simulink model "hand_assembly_3test"  (R2024b)
settings: Solver=daessc  StartTime=0.0  StopTime=10.0  RelTol=1e-3
values from neighbouring files (symbols this model uses):
  Ix1 = 0.000555447536833    [C6_workspace.mat]
  Ix2 = 0.000647276077146    [C6_workspace.mat]
  Ix3 = 0.000647276077146    [C6_workspace.mat]
  Ix4 = 0.00061268668168    [C6_workspace.mat]
  Iy1 = 0.000281297083333    [C6_workspace.mat]
  Iy2 = 0.000285516539583    [C6_workspace.mat]
  Iy3 = 0.000285516539583    [C6_workspace.mat]
  Iy4 = 0.000286923025    [C6_workspace.mat]
  Iz1 = 0.000673203786833    [C6_workspace.mat]
  Iz2 = 0.000766798670896    [C6_workspace.mat]
  Iz3 = 0.000766798670896    [C6_workspace.mat]
  Iz4 = 0.00073279805668    [C6_workspace.mat]
  m_1 = 0.245    [C6_workspace.mat]
  m_2 = 0.275    [C6_workspace.mat]
  m_3 = 0.275    [C6_workspace.mat]
  m_4 = 0.285    [C6_workspace.mat]
undefined symbols (not defined in the file or in its folder): X, Y, Z
libraries: sm_lib x115, nesl_utility x25, robotcorelib x3
(part 7 of 8)

== matlab function hand_assembly_3test/Dynamics finger 3 ==
  data: theta input size=[4,1]; tau output size=[4,1]; thetad input size=[4,1]; thetadd input size=[4,1]; thetaref input size=[4,1]; thetarefd input size=[4,1]; thetarefdd input size=[4,1]; Kp input; Kd input
function tau  = dynamics(theta, thetad, thetadd, thetaref, thetarefd, thetarefdd, Kp, Kd)
%defining parameters
m_1 = 2; 
m_2 = 2.03;
m_3 = 2.03;
m_4 = 2.04;
a_1 = 0.053311;
L_2 = 0.057755;
L_3 = 0.057755;
L_4 = 0.055798;
%d_1 = 0.04288;
w_1 = 0.03460;
w_2 = 0.03460;
w_3 = 0.03460;
w_4 = 0.03460;
h_1 = 0.02215;
h_2 = 0.02215;
h_3 = 0.02215;
h_4 = 0.02215;

%defining inputs

theta_1 = theta(1);
theta_2 = theta(2);
theta_3 = theta(3);
theta_4 = theta(4);
thetad_1 = thetad(1);
thetad_2 = thetad(2);
thetad_3 = thetad(3);
thetad_4 = thetad(4);
thetad = [thetad_1; thetad_2; thetad_3; thetad_4];

thetadd_1 = thetadd(1);
thetadd_2 = thetadd(2);
thetadd_3 = thetadd(3);
thetadd_4 = thetadd(4);
thetadd = [thetadd_1; thetadd_2; thetadd_3; thetadd_4];

thetaref_1 = thetaref(1);
thetaref_2 = thetaref(2);
thetaref_3 = thetaref(3);
thetaref_4 = thetaref(4);
thetaref = [thetaref_1; thetaref_2; thetaref_3; thetaref_4];

thetarefd_1 = thetarefd(1);
thetarefd_2 = thetarefd(2);
thetarefd_3 = thetarefd(3);
thetarefd_4 = thetarefd(4);
thetarefd = [thetarefd_1; thetarefd_2; thetarefd_3; thetarefd_4];

thetarefdd_1 = thetarefdd(1);
thetarefdd_2 = thetarefdd(2);
thetarefdd_3 = thetarefdd(3);
thetarefdd_4 = thetarefdd(4);
thetarefdd = [thetarefdd_1; thetarefdd_2; thetarefdd_3; thetarefdd_4];

thetaE = thetaref - theta;
thetaEd = thetarefd - thetad;



%%%%%%%%%%%%%%%%%%%%%%%%%%%%%%%%%%%%%%%%%%%%%%%%%%%%%%%%%%%%%%%%%%%%%%%%%%%%%%%defining inertia matrix M

M11= (1/12)*m_1*(a_1^2 + h_1^2) + (1/12)*m_2*(L_2^2 + h_2^2) + m_2*(L_2*cos(theta_2) + L_3*cos(theta_2 + theta_3) + L_4*cos(theta_2 + theta_3 + theta_4) + a_1)^2*sin(theta_1)^2 + (1/12)*m_3*(L_3^2 + h_3^2) + m_3*(L_2*cos(theta_2) + L_3*cos(theta_2 + theta_3) + L_4*cos(theta_2 + theta_3 + theta_4) + a_1)^2*cos(theta_1)^2 + (1/12)*m_4*(L_4^2 + h_4^2);
M12 = -m_2*(-L_2*sin(theta_2) - L_3*sin(theta_2 + theta_3) - L_4*sin(theta_2 + theta_3 + theta_4))*(L_2*cos(theta_2) + L_3*cos(theta_2 + theta_3) + L_4*cos(theta_2 + theta_3 + theta_4) + a_1)*sin(theta_1)*cos(theta_1) + m_3*(-L_2*sin(theta_2) - L_3*sin(theta_2 + theta_3) - L_4*sin(theta_2 + theta_3 + theta_4))*(L_2*cos(theta_2) + L_3*cos(theta_2 + theta_3) + L_4*cos(theta_2 + theta_3 + theta_4) + a_1)*sin(theta_1)*cos(theta_1);

M13 = -m_2*(-L_3*sin(theta_2 + theta_3) - L_4*sin(theta_2 + theta_3 + theta_4))*(L_2*cos(theta_2) + L_3*cos(theta_2 + theta_3) + L_4*cos(theta_2 + theta_3 + theta_4) + a_1)*sin(theta_1)*cos(theta_1) + m_3*(-L_3*sin(theta_2 + theta_3) - L_4*sin(theta_2 + theta_3 + theta_4))*(L_2*cos(theta_2) + L_3*cos(theta_2 + theta_3) + L_4*cos(theta_2 + theta_3 + theta_4) + a_1)*sin(theta_1)*cos(theta_1);
M14 = L_4*m_2*(L_2*cos(theta_2) + L_3*cos(theta_2 + theta_3) + L_4*cos(theta_2 + theta_3 + theta_4) + a_1)*sin(theta_1)*sin(theta_2 + theta_3 + theta_4)*cos(theta_1) - L_4*m_3*(L_2*cos(theta_2) + L_3*cos(theta_2 + theta_3) + L_4*cos(theta_2 + theta_3 + theta_4) + a_1)*sin(theta_1)*sin(theta_2 + theta_3 + theta_4)*cos(theta_1);

M21 = -m_2*(-L_2*sin(theta_2) - L_3*sin(theta_2 + theta_3) - L_4*sin(theta_2 + theta_3 + theta_4))*(L_2*cos(theta_2) + L_3*cos(theta_2 + theta_3) + L_4*cos(theta_2 + theta_3 + theta_4) + a_1)*sin(theta_1)*cos(theta_1) + m_3*(-L_2*sin(theta_2) - L_3*sin(theta_2 + theta_3) - L_4*sin(theta_2 + theta_3 + theta_4))*(L_2*cos(theta_2) + L_3*cos(theta_2 + theta_3) + L_4*cos(theta_2 + theta_3 + theta_4) + a_1)*sin(theta_1)*cos(theta_1);
M22 = (1/12)*m_1*(a_1^2 + w_1^2) + (1/12)*m_2*(L_2^2 + w_2^2) + m_2*(-L_2*sin(theta_2) - L_3*sin(theta_2 + theta_3) - L_4*sin(theta_2 + theta_3 + theta_4))^2*cos(theta_1)^2 + (1/12)*m_3*(L_3^2 + w_3^2) + m_3*(-L_2*sin(theta_2) - L_3*sin(theta_2 + theta_3) - L_4*sin(theta_2 + theta_3 + theta_4))^2*sin(theta_1)^2 + (1/12)*m_4*(L_4^2 + w_4^2) + m_4*(L_2*cos(theta_2) + L_3*cos(theta_2 + theta_3) + L_4*cos(theta_2 + theta_3 + theta_4))^2;

M23 = (1/12)*m_1*(a_1^2 + w_1^2) + (1/12)*m_2*(L_2^2 + w_2^2) + m_2*(-L_3*sin(theta_2 + theta_3) - L_4*sin(theta_2 + theta_3 + theta_4))*(-L_2*sin(theta_2) - L_3*sin(theta_2 + theta_3) - L_4*sin(theta_2 + theta_3 + theta_4))*cos(theta_1)^2 + (1/12)*m_3*(L_3^2 + w_3^2) + m_3*(-L_3*sin(theta_2 + theta_3) - L_4*sin(theta_2 + theta_3 + theta_4))*(-L_2*sin(theta_2) - L_3*sin(theta_2 + theta_3) - L_4*sin(theta_2 + theta_3 + theta_4))*sin(theta_1)^2 + (1/12)*m_4*(L_4^2 + w_4^2) + m_4*(L_3*cos(theta_2 + theta_3) + L_4*cos(theta_2 + theta_3 + theta_4))*(L_2*cos(theta_2) + L_3*cos(theta_2 + theta_3) + L_4*cos(theta_2 + theta_3 + theta_4));
M24 = -L_4*m_2*(-L_2*sin(theta_2) - L_3*sin(theta_2 + theta_3) - L_4*sin(theta_2 + theta_3 + theta_4))*sin(theta_2 + theta_3 + theta_4)*cos(theta_1)^2 - L_4*m_3*(-L_2*sin(theta_2) - L_3*sin(theta_2 + theta_3) - L_4*sin(theta_2 + theta_3 + theta_4))*sin(theta_1)^2*sin(theta_2 + theta_3 + theta_4) + L_4*m_4*(L_2*cos(theta_2) + L_3*cos(theta_2 + theta_3) + L_4*cos(theta_2 + theta_3 + theta_4))*cos(theta_2 + theta_3 + theta_4) + (1/12)*m_1*(a_1^2 + w_1^2) + (1/12)*m_2*(L_2^2 + w_2^2) + (1/12)*m_3*(L_3^2 + w_3^2) + (1/12)*m_4*(L_4^2 + w_4^2);

M31 = -m_2*(-L_3*sin(theta_2 + theta_3) - L_4*sin(theta_2 + theta_3 + theta_4))*(L_2*cos(theta_2) + L_3*cos(theta_2 + theta_3) + L_4*cos(theta_2 + theta_3 + theta_4) + a_1)*sin(theta_1)*cos(theta_1) + m_3*(-L_3*sin(theta_2 + theta_3) - L_4*sin(theta_2 + theta_3 + theta_4))*(L_2*cos(theta_2) + L_3*cos(theta_2 + theta_3) + L_4*cos(theta_2 + theta_3 + theta_4) + a_1)*sin(theta_1)*cos(theta_1);
M32 = (1/12)*m_1*(a_1^2 + w_1^2) + (1/12)*m_2*(L_2^2 + w_2^2) + m_2*(-L_3*sin(theta_2 + theta_3) - L_4*sin(theta_2 + theta_3 + theta_4))*(-L_2*sin(theta_2) - L_3*sin(theta_2 + theta_3) - L_4*sin(theta_2 + theta_3 + theta_4))*cos(theta_1)^2 + (1/12)*m_3*(L_3^2 + w_3^2) + m_3*(-L_3*sin(theta_2 + theta_3) - L_4*sin(theta_2 + theta_3 + theta_4))*(-L_2*sin(theta_2) - L_3*sin(theta_2 + theta_3) - L_4*sin(theta_2 + theta_3 + theta_4))*sin(theta_1)^2 + (1/12)*m_4*(L_4^2 + w_4^2) + m_4*(L_3*cos(theta_2 + theta_3) + L_4*cos(theta_2 + theta_3 + theta_4))*(L_2*cos(theta_2) + L_3*cos(theta_2 + theta_3) + L_4*cos(theta_2 + theta_3 + theta_4));

M33 = (1/12)*m_1*(a_1^2 + w_1^2) + (1/12)*m_2*(L_2^2 + w_2^2) + m_2*(-L_3*sin(theta_2 + theta_3) - L_4*sin(theta_2 + theta_3 + theta_4))^2*cos(theta_1)^2 + (1/12)*m_3*(L_3^2 + w_3^2) + m_3*(-L_3*sin(theta_2 + theta_3) - L_4*sin(theta_2 + theta_3 + theta_4))^2*sin(theta_1)^2 + (1/12)*m_4*(L_4^2 + w_4^2) + m_4*(L_3*cos(theta_2 + theta_3) + L_4*cos(theta_2 + theta_3 + theta_4))^2;
M34 = -L_4*m_2*(-L_3*sin(theta_2 + theta_3) - L_4*sin(theta_2 + theta_3 + theta_4))*sin(theta_2 + theta_3 + theta_4)*cos(theta_1)^2 - L_4*m_3*(-L_3*sin(theta_2 + theta_3) - L_4*sin(theta_2 + theta_3 + theta_4))*sin(theta_1)^2*sin(theta_2 + theta_3 + theta_4) + L_4*m_4*(L_3*cos(theta_2 + theta_3) + L_4*cos(theta_2 + theta_3 + theta_4))*cos(theta_2 + theta_3 + theta_4) + (1/12)*m_1*(a_1^2 + w_1^2) + (1/12)*m_2*(L_2^2 + w_2^2) + (1/12)*m_3*(L_3^2 + w_3^2) + (1/12)*m_4*(L_4^2 + w_4^2);

M41 = L_4*m_2*(L_2*cos(theta_2) + L_3*cos(theta_2 + theta_3) + L_4*cos(theta_2 + theta_3 + theta_4) + a_1)*sin(theta_1)*sin(theta_2 + theta_3 + theta_4)*cos(theta_1) - L_4*m_3*(L_2*cos(theta_2) + L_3*cos(theta_2 + theta_3) + L_4*cos(theta_2 + theta_3 + theta_4) + a_1)*sin(theta_1)*sin(theta_2 + theta_3 + theta_4)*cos(theta_1);
M42 = -L_4*m_2*(-L_2*sin(theta_2) - L_3*sin(theta_2 + theta_3) - L_4*sin(theta_2 + theta_3 + theta_4))*sin(theta_2 + theta_3 + theta_4)*cos(theta_1)^2 - L_4*m_3*(-L_2*sin(theta_2) - L_3*sin(theta_2 + theta_3) - L_4*sin(theta_2 + theta_3 + theta_4))*sin(theta_1)^2*sin(theta_2 + theta_3 + theta_4) + L_4*m_4*(L_2*cos(theta_2) + L_3*cos(theta_2 + theta_3) + L_4*cos(theta_2 + theta_3 + theta_4))*cos(theta_2 + theta_3 + theta_4) + (1/12)*m_1*(a_1^2 + w_1^2) + (1/12)*m_2*(L_2^2 + w_2^2) + (1/12)*m_3*(L_3^2 + w_3^2) + (1/12)*m_4*(L_4^2 + w_4^2);

M43 = -L_4*m_2*(-L_3*sin(theta_2 + theta_3) - L_4*sin(theta_2 + theta_3 + theta_4))*sin(theta_2 + theta_3 + theta_4)*cos(theta_1)^2 - L_4*m_3*(-L_3*sin(theta_2 + theta_3) - L_4*sin(theta_2 + theta_3 + theta_4))*sin(theta_1)^2*sin(theta_2 + theta_3 + theta_4) + L_4*m_4*(L_3*cos(theta_2 + theta_3) + L_4*cos(theta_2 + theta_3 + theta_4))*cos(theta_2 + theta_3 + theta_4) + (1/12)*m_1*(a_1^2 + w_1^2) + (1/12)*m_2*(L_2^2 + w_2^2) + (1/12)*m_3*(L_3^2 + w_3^2) + (1/12)*m_4*(L_4^2 + w_4^2);
M44 = L_4^2*m_2*sin(theta_2 + theta_3 + theta_4)^2*cos(theta_1)^2 + L_4^2*m_3*sin(theta_1)^2*sin(theta_2 + theta_3 + theta_4)^2 + L_4^2*m_4*cos(theta_2 + theta_3 + theta_4)^2 + (1/12)*m_1*(a_1^2 + w_1^2) + (1/12)*m_2*(L_2^2 + w_2^2) + (1/12)*m_3*(L_3^2 + w_3^2) + (1/12)*m_4*(L_4^2 + w_4^2);


M = [M11 M12 M13 M14;...
    M21 M22 M23 M24; ...
    M31 M32 M33 M34; ...
    M41 M42 M43 M44];


% %%%%%%%%%%%%%%%%%%%%%%%%%%%%%%%%%%%%%%%%%%%%%%%%%%%%%%%%%%%%%%%%%%%%%%%%%%%%%%%%%%%%%%%%%%%%%%%%%%%%%%%%%defining the Coriolis matrix C

C11 = thetad_1*(1.0*m_2*(L_2*cos(theta_2) + L_3*cos(theta_2 + theta_3) + L_4*cos(theta_2 + theta_3 + theta_4) + a_1)^2*sin(theta_1)*cos(theta_1) - 1.0*m_3*(L_2*cos(theta_2) + L_3*cos(theta_2 + theta_3) + L_4*cos(theta_2 + theta_3 + theta_4) + a_1)^2*sin(theta_1)*cos(theta_1)) + thetad_2*(0.5*m_2*(-2*L_2*sin(theta_2) - 2*L_3*sin(theta_2 + theta_3) - 2*L_4*sin(theta_2 + theta_3 + theta_4))*(L_2*cos(theta_2) + L_3*cos(theta_2 + theta_3) + L_4*cos(theta_2 + theta_3 + theta_4) + a_1)*sin(theta_1)^2 + 0.5*m_3*(-2*L_2*sin(theta_2) - 2*L_3*sin(theta_2 + theta_3) - 2*L_4*sin(theta_2 + theta_3 + theta_4))*(L_2*cos(theta_2) + L_3*cos(theta_2 + theta_3) + L_4*cos(theta_2 + theta_3 + theta_4) + a_1)*cos(theta_1)^2) + thetad_3*(0.5*m_2*(-2*L_3*sin(theta_2 + theta_3) - 2*L_4*sin(theta_2 + theta_3 + theta_4))*(L_2*cos(theta_2) + L_3*cos(theta_2 + theta_3) + L_4*cos(theta_2 + theta_3 + theta_4) + a_1)*sin(theta_1)^2 + 0.5*m_3*(-2*L_3*sin(theta_2 + theta_3) - 2*L_4*sin(theta_2 + theta_3 + theta_4))*(L_2*cos(theta_2) + L_3*cos(theta_2 + theta_3) + L_4*cos(theta_2 + theta_3 + theta_4) + a_1)*cos(theta_1)^2) + thetad_4*(-1.0*L_4*m_2*(L_2*cos(theta_2) + L_3*cos(theta_2 + theta_3) + L_4*cos(theta_2 + theta_3 + theta_4) + a_1)*sin(theta_1)^2*sin(theta_2 + theta_3 + theta_4) - 1.0*L_4*m_3*(L_2*cos(theta_2) + L_3*cos(theta_2 + theta_3) + L_4*cos(theta_2 + theta_3 + theta_4) + a_1)*sin(theta_2 + theta_3 + theta_4)*cos(theta_1)^2);
C12 = thetad_1*(0.5*m_2*(-2*L_2*sin(theta_2) - 2*L_3*sin(theta_2 + theta_3) - 2*L_4*sin(theta_2 + theta_3 + theta_4))*(L_2*cos(theta_2) + L_3*cos(theta_2 + theta_3) + L_4*cos(theta_2 + theta_3 + theta_4) + a_1)*sin(theta_1)^2 + 0.5*m_3*(-2*L_2*sin(theta_2) - 2*L_3*sin(theta_2 + theta_3) - 2*L_4*sin(theta_2 + theta_3 + theta_4))*(L_2*cos(theta_2) + L_3*cos(theta_2 + theta_3) + L_4*cos(theta_2 + theta_3 + theta_4) + a_1)*cos(theta_1)^2) + thetad_2*(-1.0*m_2*(-L_2*cos(theta_2) - L_3*cos(theta_2 + theta_3) - L_4*cos(theta_2 + theta_3 + theta_4))*(L_2*cos(theta_2) + L_3*cos(theta_2 + theta_3) + L_4*cos(theta_2 + theta_3 + theta_4) + a_1)*sin(theta_1)*cos(theta_1) + 1.0*m_3*(-L_2*cos(theta_2) - L_3*cos(theta_2 + theta_3) - L_4*cos(theta_2 + theta_3 + theta_4))*(L_2*cos(theta_2) + L_3*cos(theta_2 + theta_3) + L_4*cos(theta_2 + theta_3 + theta_4) + a_1)*sin(theta_1)*cos(theta_1)) + thetad_3*(-1.0*m_2*(-L_3*cos(theta_2 + theta_3) - L_4*cos(theta_2 + theta_3 + theta_4))*(L_2*cos(theta_2) + L_3*cos(theta_2 + theta_3) + L_4*cos(theta_2 + theta_3 + theta_4) + a_1)*sin(theta_1)*cos(theta_1) + 1.0*m_3*(-L_3*cos(theta_2 + theta_3) - L_4*cos(theta_2 + theta_3 + theta_4))*(L_2*cos(theta_2) + L_3*cos(theta_2 + theta_3) + L_4*cos(theta_2 + theta_3 + theta_4) + a_1)*sin(theta_1)*cos(theta_1)) + thetad_4*(1.0*L_4*m_2*(L_2*cos(theta_2) + L_3*cos(theta_2 + theta_3) + L_4*cos(theta_2 + theta_3 + theta_4) + a_1)*sin(theta_1)*cos(theta_1)*cos(theta_2 + theta_3 + theta_4) - 1.0*L_4*m_3*(L_2*cos(theta_2) + L_3*cos(theta_2 + theta_3) + L_4*cos(theta_2 + theta_3 + theta_4) + a_1)*sin(theta_1)*cos(theta_1)*cos(theta_2 + theta_3 + theta_4));
C13 = thetad_1*(0.5*m_2*(-2*L_3*sin(theta_2 + theta_3) - 2*L_4*sin(theta_2 + theta_3 + theta_4))*(L_2*cos(theta_2) + L_3*cos(theta_2 + theta_3) + L_4*cos(theta_2 + theta_3 + theta_4) + a_1)*sin(theta_1)^2 + 0.5*m_3*(-2*L_3*sin(theta_2 + theta_3) - 2*L_4*sin(theta_2 + theta_3 + theta_4))*(L_2*cos(theta_2) + L_3*cos(theta_2 + theta_3) + L_4*cos(theta_2 + theta_3 + theta_4) + a_1)*cos(theta_1)^2) + thetad_2*(-1.0*m_2*(-L_3*cos(theta_2 + theta_3) - L_4*cos(theta_2 + theta_3 + theta_4))*(L_2*cos(theta_2) + L_3*cos(theta_2 + theta_3) + L_4*cos(theta_2 + theta_3 + theta_4) + a_1)*sin(theta_1)*cos(theta_1) + 1.0*m_3*(-L_3*cos(theta_2 + theta_3) - L_4*cos(theta_2 + theta_3 + theta_4))*(L_2*cos(theta_2) + L_3*cos(theta_2 + theta_3) + L_4*cos(theta_2 + theta_3 + theta_4) + a_1)*sin(theta_1)*cos(theta_1)) + thetad_3*(-1.0*m_2*(-L_3*cos(theta_2 + theta_3) - L_4*cos(theta_2 + theta_3 + theta_4))*(L_2*cos(theta_2) + L_3*cos(theta_2 + theta_3) + L_4*cos(theta_2 + theta_3 + theta_4) + a_1)*sin(theta_1)*cos(theta_1) + 1.0*m_3*(-L_3*cos(theta_2 + theta_3) - L_4*cos(theta_2 + theta_3 + theta_4))*(L_2*cos(theta_2) + L_3*cos(theta_2 + theta_3) + L_4*cos(theta_2 + theta_3 + theta_4) + a_1)*sin(theta_1)*cos(theta_1)) + thetad_4*(1.0*L_4*m_2*(L_2*cos(theta_2) + L_3*cos(theta_2 + theta_3) + L_4*cos(theta_2 + theta_3 + theta_4) + a_1)*sin(theta_1)*cos(theta_1)*cos(theta_2 + theta_3 + theta_4) - 1.0*L_4*m_3*(L_2*cos(theta_2) + L_3*cos(theta_2 + theta_3) + L_4*cos(theta_2 + theta_3 + theta_4) + a_1)*sin(theta_1)*cos(theta_1)*cos(theta_2 + theta_3 + theta_4));
C14 = thetad_1*(-1.0*L_4*m_2*(L_2*cos(theta_2) + L_3*cos(theta_2 + theta_3) + L_4*cos(theta_2 + theta_3 + theta_4) + a_1)*sin(theta_1)^2*sin(theta_2 + theta_3 + theta_4) - 1.0*L_4*m_3*(L_2*cos(theta_2) + L_3*cos(theta_2 + theta_3) + L_4*cos(theta_2 + theta_3 + theta_4) + a_1)*sin(theta_2 + theta_3 + theta_4)*cos(theta_1)^2) + thetad_2*(1.0*L_4*m_2*(L_2*cos(theta_2) + L_3*cos(theta_2 + theta_3) + L_4*cos(theta_2 + theta_3 + theta_4) + a_1)*sin(theta_1)*cos(theta_1)*cos(theta_2 + theta_3 + theta_4) - 1.0*L_4*m_3*(L_2*cos(theta_2) + L_3*cos(theta_2 + theta_3) + L_4*cos(theta_2 + theta_3 + theta_4) + a_1)*sin(theta_1)*cos(theta_1)*cos(theta_2 + theta_3 + theta_4)) + thetad_3*(1.0*L_4*m_2*(L_2*cos(theta_2) + L_3*cos(theta_2 + theta_3) + L_4*cos(theta_2 + theta_3 + theta_4) + a_1)*sin(theta_1)*cos(theta_1)*cos(theta_2 + theta_3 + theta_4) - 1.0*L_4*m_3*(L_2*cos(theta_2) + L_3*cos(theta_2 + theta_3) + L_4*cos(theta_2 + theta_3 + theta_4) + a_1)*sin(theta_1)*cos(theta_1)*cos(theta_2 + theta_3 + theta_4)) + thetad_4*(1.0*L_4*m_2*(L_2*cos(theta_2) + L_3*cos(theta_2 + theta_3) + L_4*cos(theta_2 + theta_3 + theta_4) + a_1)*sin(theta_1)*cos(theta_1)*cos(theta_2 + theta_3 + theta_4) - 1.0*L_4*m_3*(L_2*cos(theta_2) + L_3*cos(theta_2 + theta_3) + L_4*cos(theta_2 + theta_3 + theta_4) + a_1)*sin(theta_1)*cos(theta_1)*cos(theta_2 + theta_3 + theta_4));

C21 = thetad_1*(-0.5*m_2*(-2*L_2*sin(theta_2) - 2*L_3*sin(theta_2 + theta_3) - 2*L_4*sin(theta_2 + theta_3 + theta_4))*(L_2*cos(theta_2) + L_3*cos(theta_2 + theta_3) + L_4*cos(theta_2 + theta_3 + theta_4) + a_1)*sin(theta_1)^2 + 1.0*m_2*(-L_2*sin(theta_2) - L_3*sin(theta_2 + theta_3) - L_4*sin(theta_2 + theta_3 + theta_4))*(L_2*cos(theta_2) + L_3*cos(theta_2 + theta_3) + L_4*cos(theta_2 + theta_3 + theta_4) + a_1)*sin(theta_1)^2 - 1.0*m_2*(-L_2*sin(theta_2) - L_3*sin(theta_2 + theta_3) - L_4*sin(theta_2 + theta_3 + theta_4))*(L_2*cos(theta_2) + L_3*cos(theta_2 + theta_3) + L_4*cos(theta_2 + theta_3 + theta_4) + a_1)*cos(theta_1)^2 - 0.5*m_3*(-2*L_2*sin(theta_2) - 2*L_3*sin(theta_2 + theta_3) - 2*L_4*sin(theta_2 + theta_3 + theta_4))*(L_2*cos(theta_2) + L_3*cos(theta_2 + theta_3) + L_4*cos(theta_2 + theta_3 + theta_4) + a_1)*cos(theta_1)^2 - 1.0*m_3*(-L_2*sin(theta_2) - L_3*sin(theta_2 + theta_3) - L_4*sin(theta_2 + theta_3 + theta_4))*(L_2*cos(theta_2) + L_3*cos(theta_2 + theta_3) + L_4*cos(theta_2 + theta_3 + theta_4) + a_1)*sin(theta_1)^2 + 1.0*m_3*(-L_2*sin(theta_2) - L_3*sin(theta_2 + theta_3) - L_4*sin(theta_2 + theta_3 + theta_4))*(L_2*cos(theta_2) + L_3*cos(theta_2 + theta_3) + L_4*cos(theta_2 + theta_3 + theta_4) + a_1)*cos(theta_1)^2) + thetad_2*(-1.0*m_2*(-L_2*sin(theta_2) - L_3*sin(theta_2 + theta_3) - L_4*sin(theta_2 + theta_3 + theta_4))^2*sin(theta_1)*cos(theta_1) + 1.0*m_3*(-L_2*sin(theta_2) - L_3*sin(theta_2 + theta_3) - L_4*sin(theta_2 + theta_3 + theta_4))^2*sin(theta_1)*cos(theta_1)) + thetad_3*(-1.0*m_2*(-L_3*sin(theta_2 + theta_3) - L_4*sin(theta_2 + theta_3 + theta_4))*(-L_2*sin(theta_2) - L_3*sin(theta_2 + theta_3) - L_4*sin(theta_2 + theta_3 + theta_4))*sin(theta_1)*cos(theta_1) + 1.0*m_3*(-L_3*sin(theta_2 + theta_3) - L_4*sin(theta_2 + theta_3 + theta_4))*(-L_2*sin(theta_2) - L_3*sin(theta_2 + theta_3) - L_4*sin(theta_2 + theta_3 + theta_4))*sin(theta_1)*cos(theta_1)) + thetad_4*(1.0*L_4*m_2*(-L_2*sin(theta_2) - L_3*sin(theta_2 + theta_3) - L_4*sin(theta_2 + theta_3 + theta_4))*sin(theta_1)*sin(theta_2 + theta_3 + theta_4)*cos(theta_1) - 1.0*L_4*m_3*(-L_2*sin(theta_2) - L_3*sin(theta_2 + theta_3) - L_4*sin(theta_2 + theta_3 + theta_4))*sin(theta_1)*sin(theta_2 + theta_3 + theta_4)*cos(theta_1));
C22 = thetad_1*(-1.0*m_2*(-L_2*sin(theta_2) - L_3*sin(theta_2 + theta_3) - L_4*sin(theta_2 + theta_3 + theta_4))^2*sin(theta_1)*cos(theta_1) + 1.0*m_3*(-L_2*sin(theta_2) - L_3*sin(theta_2 + theta_3) - L_4*sin(theta_2 + theta_3 + theta_4))^2*sin(theta_1)*cos(theta_1)) + thetad_2*(0.5*m_2*(-L_2*sin(theta_2) - L_3*sin(theta_2 + theta_3) - L_4*sin(theta_2 + theta_3 + theta_4))*(-2*L_2*cos(theta_2) - 2*L_3*cos(theta_2 + theta_3) - 2*L_4*cos(theta_2 + theta_3 + theta_4))*cos(theta_1)^2 + 0.5*m_3*(-L_2*sin(theta_2) - L_3*sin(theta_2 + theta_3) - L_4*sin(theta_2 + theta_3 + theta_4))*(-2*L_2*cos(theta_2) - 2*L_3*cos(theta_2 + theta_3) - 2*L_4*cos(theta_2 + theta_3 + theta_4))*sin(theta_1)^2 + 0.5*m_4*(-2*L_2*sin(theta_2) - 2*L_3*sin(theta_2 + theta_3) - 2*L_4*sin(theta_2 + theta_3 + theta_4))*(L_2*cos(theta_2) + L_3*cos(theta_2 + theta_3) + L_4*cos(theta_2 + theta_3 + theta_4))) + thetad_3*(0.5*m_2*(-2*L_3*cos(theta_2 + theta_3) - 2*L_4*cos(theta_2 + theta_3 + theta_4))*(-L_2*sin(theta_2) - L_3*sin(theta_2 + theta_3) - L_4*sin(theta_2 + theta_3 + theta_4))*cos(theta_1)^2 + 0.5*m_3*(-2*L_3*cos(theta_2 + theta_3) - 2*L_4*cos(theta_2 + theta_3 + theta_4))*(-L_2*sin(theta_2) - L_3*sin(theta_2 + theta_3) - L_4*sin(theta_2 + theta_3 + theta_4))*sin(theta_1)^2 + 0.5*m_4*(-2*L_3*sin(theta_2 + theta_3) - 2*L_4*sin(theta_2 + theta_3 + theta_4))*(L_2*cos(theta_2) + L_3*cos(theta_2 + theta_3) + L_4*cos(theta_2 + theta_3 + theta_4))) + thetad_4*(-1.0*L_4*m_2*(-L_2*sin(theta_2) - L_3*sin(theta_2 + theta_3) - L_4*sin(theta_2 + theta_3 + theta_4))*cos(theta_1)^2*cos(theta_2 + theta_3 + theta_4) - 1.0*L_4*m_3*(-L_2*sin(theta_2) - L_3*sin(theta_2 + theta_3) - L_4*sin(theta_2 + theta_3 + theta_4))*sin(theta_1)^2*cos(theta_2 + theta_3 + theta_4) - 1.0*L_4*m_4*(L_2*cos(theta_2) + L_3*cos(theta_2 + theta_3) + L_4*cos(theta_2 + theta_3 + theta_4))*sin(theta_2 + theta_3 + theta_4));
C23 = thetad_1*(-1.0*m_2*(-L_3*sin(theta_2 + theta_3) - L_4*sin(theta_2 + theta_3 + theta_4))*(-L_2*sin(theta_2) - L_3*sin(theta_2 + theta_3) - L_4*sin(theta_2 + theta_3 + theta_4))*sin(theta_1)*cos(theta_1) + 1.0*m_3*(-L_3*sin(theta_2 + theta_3) - L_4*sin(theta_2 + theta_3 + theta_4))*(-L_2*sin(theta_2) - L_3*sin(theta_2 + theta_3) - L_4*sin(theta_2 + theta_3 + theta_4))*sin(theta_1)*cos(theta_1)) + thetad_2*(0.5*m_2*(-2*L_3*cos(theta_2 + theta_3) - 2*L_4*cos(theta_2 + theta_3 + theta_4))*(-L_2*sin(theta_2) - L_3*sin(theta_2 + theta_3) - L_4*sin(theta_2 + theta_3 + theta_4))*cos(theta_1)^2 + 0.5*m_3*(-2*L_3*cos(theta_2 + theta_3) - 2*L_4*cos(theta_2 + theta_3 + theta_4))*(-L_2*sin(theta_2) - L_3*sin(theta_2 + theta_3) - L_4*sin(theta_2 + theta_3 + theta_4))*sin(theta_1)^2 + 0.5*m_4*(-2*L_3*sin(theta_2 + theta_3) - 2*L_4*sin(theta_2 + theta_3 + theta_4))*(L_2*cos(theta_2) + L_3*cos(theta_2 + theta_3) + L_4*cos(theta_2 + theta_3 + theta_4))) + thetad_3*(-0.5*m_2*(-L_3*sin(theta_2 + theta_3) - L_4*sin(theta_2 + theta_3 + theta_4))*(-2*L_3*cos(theta_2 + theta_3) - 2*L_4*cos(theta_2 + theta_3 + theta_4))*cos(theta_1)^2 + 1.0*m_2*(-L_3*sin(theta_2 + theta_3) - L_4*sin(theta_2 + theta_3 + theta_4))*(-L_3*cos(theta_2 + theta_3) - L_4*cos(theta_2 + theta_3 + theta_4))*cos(theta_1)^2 + 1.0*m_2*(-L_3*cos(theta_2 + theta_3) - L_4*cos(theta_2 + theta_3 + theta_4))*(-L_2*sin(theta_2) - L_3*sin(theta_2 + theta_3) - L_4*sin(theta_2 + theta_3 + theta_4))*cos(theta_1)^2 - 0.5*m_3*(-L_3*sin(theta_2 + theta_3) - L_4*sin(theta_2 + theta_3 + theta_4))*(-2*L_3*cos(theta_2 + theta_3) - 2*L_4*cos(theta_2 + theta_3 + theta_4))*sin(theta_1)^2 + 1.0*m_3*(-L_3*sin(theta_2 + theta_3) - L_4*sin(theta_2 + theta_3 + theta_4))*(-L_3*cos(theta_2 + theta_3) - L_4*cos(theta_2 + theta_3 + theta_4))*sin(theta_1)^2 + 1.0*m_3*(-L_3*cos(theta_2 + theta_3) - L_4*cos(theta_2 + theta_3 + theta_4))*(-L_2*sin(theta_2) - L_3*sin(theta_2 + theta_3) - L_4*sin(theta_2 + theta_3 + theta_4))*sin(theta_1)^2 - 0.5*m_4*(-2*L_3*sin(theta_2 + theta_3) - 2*L_4*sin(theta_2 + theta_3 + theta_4))*(L_3*cos(theta_2 + theta_3) + L_4*cos(theta_2 + theta_3 + theta_4)) + 1.0*m_4*(-L_3*sin(theta_2 + theta_3) - L_4*sin(theta_2 + theta_3 + theta_4))*(L_3*cos(theta_2 + theta_3) + L_4*cos(theta_2 + theta_3 + theta_4)) + 1.0*m_4*(-L_3*sin(theta_2 + theta_3) - L_4*sin(theta_2 + theta_3 + theta_4))*(L_2*cos(theta_2) + L_3*cos(theta_2 + theta_3) + L_4*cos(theta_2 + theta_3 + theta_4))) + thetad_4*(-1.0*L_4*m_2*(-L_2*sin(theta_2) - L_3*sin(theta_2 + theta_3) - L_4*sin(theta_2 + theta_3 + theta_4))*cos(theta_1)^2*cos(theta_2 + theta_3 + theta_4) - 1.0*L_4*m_3*(-L_2*sin(theta_2) - L_3*sin(theta_2 + theta_3) - L_4*sin(theta_2 + theta_3 + theta_4))*sin(theta_1)^2*cos(theta_2 + theta_3 + theta_4) - 1.0*L_4*m_4*(L_2*cos(theta_2) + L_3*cos(theta_2 + theta_3) + L_4*cos(theta_2 + theta_3 + theta_4))*sin(theta_2 + theta_3 + theta_4));
C24 = thetad_1*(-1.0*m_2*(-L_3*sin(theta_2 + theta_3) - L_4*sin(theta_2 + theta_3 + theta_4))^2*sin(theta_1)*cos(theta_1) + 1.0*m_3*(-L_3*sin(theta_2 + theta_3) - L_4*sin(theta_2 + theta_3 + theta_4))^2*sin(theta_1)*cos(theta_1)) + thetad_2*(0.5*m_2*(-L_3*sin(theta_2 + theta_3) - L_4*sin(theta_2 + theta_3 + theta_4))*(-2*L_3*cos(theta_2 + theta_3) - 2*L_4*cos(theta_2 + theta_3 + theta_4))*cos(theta_1)^2 + 0.5*m_3*(-L_3*sin(theta_2 + theta_3) - L_4*sin(theta_2 + theta_3 + theta_4))*(-2*L_3*cos(theta_2 + theta_3) - 2*L_4*cos(theta_2 + theta_3 + theta_4))*sin(theta_1)^2 + 0.5*m_4*(-2*L_3*sin(theta_2 + theta_3) - 2*L_4*sin(theta_2 + theta_3 + theta_4))*(L_3*cos(theta_2 + theta_3) + L_4*cos(theta_2 + theta_3 + theta_4))) + thetad_3*(0.5*m_2*(-L_3*sin(theta_2 + theta_3) - L_4*sin(theta_2 + theta_3 + theta_4))*(-2*L_3*cos(theta_2 + theta_3) - 2*L_4*cos(theta_2 + theta_3 + theta_4))*cos(theta_1)^2 + 0.5*m_3*(-L_3*sin(theta_2 + theta_3) - L_4*sin(theta_2 + theta_3 + theta_4))*(-2*L_3*cos(theta_2 + theta_3) - 2*L_4*cos(theta_2 + theta_3 + theta_4))*sin(theta_1)^2 + 0.5*m_4*(-2*L_3*sin(theta_2 + theta_3) - 2*L_4*sin(theta_2 + theta_3 + theta_4))*(L_3*cos(theta_2 + theta_3) + L_4*cos(theta_2 + theta_3 + theta_4))) + thetad_4*(-1.0*L_4*m_2*(-L_3*sin(theta_2 + theta_3) - L_4*sin(theta_2 + theta_3 + theta_4))*cos(theta_1)^2*cos(theta_2 + theta_3 + theta_4) - 1.0*L_4*m_3*(-L_3*sin(theta_2 + theta_3) - L_4*sin(theta_2 + theta_3 + theta_4))*sin(theta_1)^2*cos(theta_2 + theta_3 + theta_4) - 1.0*L_4*m_4*(L_3*cos(theta_2 + theta_3) + L_4*cos(theta_2 + theta_3 + theta_4))*sin(theta_2 + theta_3 + theta_4));

C31 = thetad_1*(-0.5*m_2*(-2*L_3*sin(theta_2 + theta_3) - 2*L_4*sin(theta_2 + theta_3 + theta_4))*(L_2*cos(theta_2) + L_3*cos(theta_2 + theta_3) + L_4*cos(theta_2 + theta_3 + theta_4) + a_1)*sin(theta_1)^2 + 1.0*m_2*(-L_3*sin(theta_2 + theta_3) - L_4*sin(theta_2 + theta_3 + theta_4))*(L_2*cos(theta_2) + L_3*cos(theta_2 + theta_3) + L_4*cos(theta_2 + theta_3 + theta_4) + a_1)*sin(theta_1)^2 - 1.0*m_2*(-L_3*sin(theta_2 + theta_3) - L_4*sin(theta_2 + theta_3 + theta_4))*(L_2*cos(theta_2) + L_3*cos(theta_2 + theta_3) + L_4*cos(theta_2 + theta_3 + theta_4) + a_1)*cos(theta_1)^2 - 0.5*m_3*(-2*L_3*sin(theta_2 + theta_3) - 2*L_4*sin(theta_2 + theta_3 + theta_4))*(L_2*cos(theta_2) + L_3*cos(theta_2 + theta_3) + L_4*cos(theta_2 + theta_3 + theta_4) + a_1)*cos(theta_1)^2 - 1.0*m_3*(-L_3*sin(theta_2 + theta_3) - L_4*sin(theta_2 + theta_3 + theta_4))*(L_2*cos(theta_2) + L_3*cos(theta_2 + theta_3) + L_4*cos(theta_2 + theta_3 + theta_4) + a_1)*sin(theta_1)^2 + 1.0*m_3*(-L_3*sin(theta_2 + theta_3) - L_4*sin(theta_2 + theta_3 + theta_4))*(L_2*cos(theta_2) + L_3*cos(theta_2 + theta_3) + L_4*cos(theta_2 + theta_3 + theta_4) + a_1)*cos(theta_1)^2) + thetad_2*(-1.0*m_2*(-L_3*sin(theta_2 + theta_3) - L_4*sin(theta_2 + theta_3 + theta_4))*(-L_2*sin(theta_2) - L_3*sin(theta_2 + theta_3) - L_4*sin(theta_2 + theta_3 + theta_4))*sin(theta_1)*cos(theta_1) + 1.0*m_3*(-L_3*sin(theta_2 + theta_3) - L_4*sin(theta_2 + theta_3 + theta_4))*(-L_2*sin(theta_2) - L_3*sin(theta_2 + theta_3) - L_4*sin(theta_2 + theta_3 + theta_4))*sin(theta_1)*cos(theta_1)) + thetad_3*(-1.0*m_2*(-L_3*sin(theta_2 + theta_3) - L_4*sin(theta_2 + theta_3 + theta_4))^2*sin(theta_1)*cos(theta_1) + 1.0*m_3*(-L_3*sin(theta_2 + theta_3) - L_4*sin(theta_2 + theta_3 + theta_4))^2*sin(theta_1)*cos(theta_1)) + thetad_4*(1.0*L_4*m_2*(-L_3*sin(theta_2 + theta_3) - L_4*sin(theta_2 + theta_3 + theta_4))*sin(theta_1)*sin(theta_2 + theta_3 + theta_4)*cos(theta_1) - 1.0*L_4*m_3*(-L_3*sin(theta_2 + theta_3) - L_4*sin(theta_2 + theta_3 + theta_4))*sin(theta_1)*sin(theta_2 + theta_3 + theta_4)*cos(theta_1));
C32 = thetad_1*(-1.0*m_2*(-L_3*sin(theta_2 + theta_3) - L_4*sin(theta_2 + theta_3 + theta_4))*(-L_2*sin(theta_2) - L_3*sin(theta_2 + theta_3) - L_4*sin(theta_2 + theta_3 + theta_4))*sin(theta_1)*cos(theta_1) + 1.0*m_3*(-L_3*sin(theta_2 + theta_3) - L_4*sin(theta_2 + theta_3 + theta_4))*(-L_2*sin(theta_2) - L_3*sin(theta_2 + theta_3) - L_4*sin(theta_2 + theta_3 + theta_4))*sin(theta_1)*cos(theta_1)) + thetad_2*(1.0*m_2*(-L_3*sin(theta_2 + theta_3) - L_4*sin(theta_2 + theta_3 + theta_4))*(-L_2*cos(theta_2) - L_3*cos(theta_2 + theta_3) - L_4*cos(theta_2 + theta_3 + theta_4))*cos(theta_1)^2 - 0.5*m_2*(-2*L_3*cos(theta_2 + theta_3) - 2*L_4*cos(theta_2 + theta_3 + theta_4))*(-L_2*sin(theta_2) - L_3*sin(theta_2 + theta_3) - L_4*sin(theta_2 + theta_3 + theta_4))*cos(theta_1)^2 + 1.0*m_2*(-L_3*cos(theta_2 + theta_3) - L_4*cos(theta_2 + theta_3 + theta_4))*(-L_2*sin(theta_2) - L_3*sin(theta_2 + theta_3) - L_4*sin(theta_2 + theta_3 + theta_4))*cos(theta_1)^2 + 1.0*m_3*(-L_3*sin(theta_2 + theta_3) - L_4*sin(theta_2 + theta_3 + theta_4))*(-L_2*cos(theta_2) - L_3*cos(theta_2 + theta_3) - L_4*cos(theta_2 + theta_3 + theta_4))*sin(theta_1)^2 - 0.5*m_3*(-2*L_3*cos(theta_2 + theta_3) - 2*L_4*cos(theta_2 + theta_3 + theta_4))*(-L_2*sin(theta_2) - L_3*sin(theta_2 + theta_3) - L_4*sin(theta_2 + theta_3 + theta_4))*sin(theta_1)^2 + 1.0*m_3*(-L_3*cos(theta_2 + theta_3) - L_4*cos(theta_2 + theta_3 + theta_4))*(-L_2*sin(theta_2) - L_3*sin(theta_2 + theta_3) - L_4*sin(theta_2 + theta_3 + theta_4))*sin(theta_1)^2 - 0.5*m_4*(-2*L_3*sin(theta_2 + theta_3) - 2*L_4*sin(theta_2 + theta_3 + theta_4))*(L_2*cos(theta_2) + L_3*cos(theta_2 + theta_3) + L_4*cos(theta_2 + theta_3 + theta_4)) + 1.0*m_4*(-L_3*sin(theta_2 + theta_3) - L_4*sin(theta_2 + theta_3 + theta_4))*(L_2*cos(theta_2) + L_3*cos(theta_2 + theta_3) + L_4*cos(theta_2 + theta_3 + theta_4)) + 1.0*m_4*(L_3*cos(theta_2 + theta_3) + L_4*cos(theta_2 + theta_3 + theta_4))*(-L_2*sin(theta_2) - L_3*sin(theta_2 + theta_3) - L_4*sin(theta_2 + theta_3 + theta_4))) + thetad_3*(0.5*m_2*(-L_3*sin(theta_2 + theta_3) - L_4*sin(theta_2 + theta_3 + theta_4))*(-2*L_3*cos(theta_2 + theta_3) - 2*L_4*cos(theta_2 + theta_3 + theta_4))*cos(theta_1)^2 + 0.5*m_3*(-L_3*sin(theta_2 + theta_3) - L_4*sin(theta_2 + theta_3 + theta_4))*(-2*L_3*cos(theta_2 + theta_3) - 2*L_4*cos(theta_2 + theta_3 + theta_4))*sin(theta_1)^2 + 0.5*m_4*(-2*L_3*sin(theta_2 + theta_3) - 2*L_4*sin(theta_2 + theta_3 + theta_4))*(L_3*cos(theta_2 + theta_3) + L_4*cos(theta_2 + theta_3 + theta_4))) + thetad_4*(-1.0*L_4*m_2*(-L_3*sin(theta_2 + theta_3) - L_4*sin(theta_2 + theta_3 + theta_4))*cos(theta_1)^2*cos(theta_2 + theta_3 + theta_4) - 1.0*L_4*m_3*(-L_3*sin(theta_2 + theta_3) - L_4*sin(theta_2 + theta_3 + theta_4))*sin(theta_1)^2*cos(theta_2 + theta_3 + theta_4) - 1.0*L_4*m_4*(L_3*cos(theta_2 + theta_3) + L_4*cos(theta_2 + theta_3 + theta_4))*sin(theta_2 + theta_3 + theta_4));
C33 = thetad_1*(-1.0*m_2*(-L_3*sin(theta_2 + theta_3) - L_4*sin(theta_2 + theta_3 + theta_4))^2*sin(theta_1)*cos(theta_1) + 1.0*m_3*(-L_3*sin(theta_2 + theta_3) - L_4*sin(theta_2 + theta_3 + theta_4))^2*sin(theta_1)*cos(theta_1)) + thetad_2*(0.5*m_2*(-L_3*sin(theta_2 + theta_3) - L_4*sin(theta_2 + theta_3 + theta_4))*(-2*L_3*cos(theta_2 + theta_3) - 2*L_4*cos(theta_2 + theta_3 + theta_4))*cos(theta_1)^2 + 0.5*m_3*(-L_3*sin(theta_2 + theta_3) - L_4*sin(theta_2 + theta_3 + theta_4))*(-2*L_3*cos(theta_2 + theta_3) - 2*L_4*cos(theta_2 + theta_3 + theta_4))*sin(theta_1)^2 + 0.5*m_4*(-2*L_3*sin(theta_2 + theta_3) - 2*L_4*sin(theta_2 + theta_3 + theta_4))*(L_3*cos(theta_2 + theta_3) + L_4*cos(theta_2 + theta_3 + theta_4))) + thetad_3*(0.5*m_2*(-L_3*sin(theta_2 + theta_3) - L_4*sin(theta_2 + theta_3 + theta_4))*(-2*L_3*cos(theta_2 + theta_3) - 2*L_4*cos(theta_2 + theta_3 + theta_4))*cos(theta_1)^2 + 0.5*m_3*(-L_3*sin(theta_2 + theta_3) - L_4*sin(theta_2 + theta_3 + theta_4))*(-2*L_3*cos(theta_2 + theta_3) - 2*L_4*cos(theta_2 + theta_3 + theta_4))*sin(theta_1)^2 + 0.5*m_4*(-2*L_3*sin(theta_2 + theta_3) - 2*L_4*sin(theta_2 + theta_3 + theta_4))*(L_3*cos(theta_2 + theta_3) + L_4*cos(theta_2 + theta_3 + theta_4))) + thetad_4*(-1.0*L_4*m_2*(-L_3*sin(theta_2 + theta_3) - L_4*sin(theta_2 + theta_3 + theta_4))*cos(theta_1)^2*cos(theta_2 + theta_3 + theta_4) - 1.0*L_4*m_3*(-L_3*sin(theta_2 + theta_3) - L_4*sin(theta_2 + theta_3 + theta_4))*sin(theta_1)^2*cos(theta_2 + theta_3 + theta_4) - 1.0*L_4*m_4*(L_3*cos(theta_2 + theta_3) + L_4*cos(theta_2 + theta_3 + theta_4))*sin(theta_2 + theta_3 + theta_4));
C34 = thetad_1*(1.0*L_4*m_2*(-L_3*sin(theta_2 + theta_3) - L_4*sin(theta_2 + theta_3 + theta_4))*sin(theta_1)*sin(theta_2 + theta_3 + theta_4)*cos(theta_1) - 1.0*L_4*m_3*(-L_3*sin(theta_2 + theta_3) - L_4*sin(theta_2 + theta_3 + theta_4))*sin(theta_1)*sin(theta_2 + theta_3 + theta_4)*cos(theta_1)) + thetad_2*(-1.0*L_4*m_2*(-L_3*sin(theta_2 + theta_3) - L_4*sin(theta_2 + theta_3 + theta_4))*cos(theta_1)^2*cos(theta_2 + theta_3 + theta_4) - 1.0*L_4*m_3*(-L_3*sin(theta_2 + theta_3) - L_4*sin(theta_2 + theta_3 + theta_4))*sin(theta_1)^2*cos(theta_2 + theta_3 + theta_4) - 1.0*L_4*m_4*(L_3*cos(theta_2 + theta_3) + L_4*cos(theta_2 + theta_3 + theta_4))*sin(theta_2 + theta_3 + theta_4)) + thetad_3*(-1.0*L_4*m_2*(-L_3*sin(theta_2 + theta_3) - L_4*sin(theta_2 + theta_3 + theta_4))*cos(theta_1)^2*cos(theta_2 + theta_3 + theta_4) - 1.0*L_4*m_3*(-L_3*sin(theta_2 + theta_3) - L_4*sin(theta_2 + theta_3 + theta_4))*sin(theta_1)^2*cos(theta_2 + theta_3 + theta_4) - 1.0*L_4*m_4*(L_3*cos(theta_2 + theta_3) + L_4*cos(theta_2 + theta_3 + theta_4))*sin(theta_2 + theta_3 + theta_4)) + thetad_4*(-1.0*L_4*m_2*(-L_3*sin(theta_2 + theta_3) - L_4*sin(theta_2 + theta_3 + theta_4))*cos(theta_1)^2*cos(theta_2 + theta_3 + theta_4) - 1.0*L_4*m_3*(-L_3*sin(theta_2 + theta_3) - L_4*sin(theta_2 + theta_3 + theta_4))*sin(theta_1)^2*cos(theta_2 + theta_3 + theta_4) - 1.0*L_4*m_4*(L_3*cos(theta_2 + theta_3) + L_4*cos(theta_2 + theta_3 + theta_4))*sin(theta_2 + theta_3 + theta_4));

C41 = thetad_1*(1.0*L_4*m_2*(L_2*cos(theta_2) + L_3*cos(theta_2 + theta_3) + L_4*cos(theta_2 + theta_3 + theta_4) + a_1)*sin(theta_2 + theta_3 + theta_4)*cos(theta_1)^2 + 1.0*L_4*m_3*(L_2*cos(theta_2) + L_3*cos(theta_2 + theta_3) + L_4*cos(theta_2 + theta_3 + theta_4) + a_1)*sin(theta_1)^2*sin(theta_2 + theta_3 + theta_4)) + thetad_2*(1.0*L_4*m_2*(-L_2*sin(theta_2) - L_3*sin(theta_2 + theta_3) - L_4*sin(theta_2 + theta_3 + theta_4))*sin(theta_1)*sin(theta_2 + theta_3 + theta_4)*cos(theta_1) - 1.0*L_4*m_3*(-L_2*sin(theta_2) - L_3*sin(theta_2 + theta_3) - L_4*sin(theta_2 + theta_3 + theta_4))*sin(theta_1)*sin(theta_2 + theta_3 + theta_4)*cos(theta_1)) + thetad_3*(1.0*L_4*m_2*(-L_3*sin(theta_2 + theta_3) - L_4*sin(theta_2 + theta_3 + theta_4))*sin(theta_1)*sin(theta_2 + theta_3 + theta_4)*cos(theta_1) - 1.0*L_4*m_3*(-L_3*sin(theta_2 + theta_3) - L_4*sin(theta_2 + theta_3 + theta_4))*sin(theta_1)*sin(theta_2 + theta_3 + theta_4)*cos(theta_1)) + thetad_4*(-1.0*L_4^2*m_2*sin(theta_1)*sin(theta_2 + theta_3 + theta_4)^2*cos(theta_1) + 1.0*L_4^2*m_3*sin(theta_1)*sin(theta_2 + theta_3 + theta_4)^2*cos(theta_1));
C42 = thetad_1*(1.0*L_4*m_2*(-L_2*sin(theta_2) - L_3*sin(theta_2 + theta_3) - L_4*sin(theta_2 + theta_3 + theta_4))*sin(theta_1)*sin(theta_2 + theta_3 + theta_4)*cos(theta_1) - 1.0*L_4*m_3*(-L_2*sin(theta_2) - L_3*sin(theta_2 + theta_3) - L_4*sin(theta_2 + theta_3 + theta_4))*sin(theta_1)*sin(theta_2 + theta_3 + theta_4)*cos(theta_1)) + thetad_2*(-1.0*L_4*m_2*(-L_2*cos(theta_2) - L_3*cos(theta_2 + theta_3) - L_4*cos(theta_2 + theta_3 + theta_4))*sin(theta_2 + theta_3 + theta_4)*cos(theta_1)^2 - 1.0*L_4*m_3*(-L_2*cos(theta_2) - L_3*cos(theta_2 + theta_3) - L_4*cos(theta_2 + theta_3 + theta_4))*sin(theta_1)^2*sin(theta_2 + theta_3 + theta_4) + 1.0*L_4*m_4*(-L_2*sin(theta_2) - L_3*sin(theta_2 + theta_3) - L_4*sin(theta_2 + theta_3 + theta_4))*cos(theta_2 + theta_3 + theta_4)) + thetad_3*(-1.0*L_4*m_2*(-L_3*cos(theta_2 + theta_3) - L_4*cos(theta_2 + theta_3 + theta_4))*sin(theta_2 + theta_3 + theta_4)*cos(theta_1)^2 - 1.0*L_4*m_3*(-L_3*cos(theta_2 + theta_3) - L_4*cos(theta_2 + theta_3 + theta_4))*sin(theta_1)^2*sin(theta_2 + theta_3 + theta_4) + 1.0*L_4*m_4*(-L_3*sin(theta_2 + theta_3) - L_4*sin(theta_2 + theta_3 + theta_4))*cos(theta_2 + theta_3 + theta_4)) + thetad_4*(1.0*L_4^2*m_2*sin(theta_2 + theta_3 + theta_4)*cos(theta_1)^2*cos(theta_2 + theta_3 + theta_4) + 1.0*L_4^2*m_3*sin(theta_1)^2*sin(theta_2 + theta_3 + theta_4)*cos(theta_2 + theta_3 + theta_4) - 1.0*L_4^2*m_4*sin(theta_2 + theta_3 + theta_4)*cos(theta_2 + theta_3 + theta_4));
C43 = thetad_1*(1.0*L_4*m_2*(-L_3*sin(theta_2 + theta_3) - L_4*sin(theta_2 + theta_3 + theta_4))*sin(theta_1)*sin(theta_2 + theta_3 + theta_4)*cos(theta_1) - 1.0*L_4*m_3*(-L_3*sin(theta_2 + theta_3) - L_4*sin(theta_2 + theta_3 + theta_4))*sin(theta_1)*sin(theta_2 + theta_3 + theta_4)*cos(theta_1)) + thetad_2*(-1.0*L_4*m_2*(-L_3*cos(theta_2 + theta_3) - L_4*cos(theta_2 + theta_3 + theta_4))*sin(theta_2 + theta_3 + theta_4)*cos(theta_1)^2 - 1.0*L_4*m_3*(-L_3*cos(theta_2 + theta_3) - L_4*cos(theta_2 + theta_3 + theta_4))*sin(theta_1)^2*sin(theta_2 + theta_3 + theta_4) + 1.0*L_4*m_4*(-L_3*sin(theta_2 + theta_3) - L_4*sin(theta_2 + theta_3 + theta_4))*cos(theta_2 + theta_3 + theta_4)) + thetad_3*(-1.0*L_4*m_2*(-L_3*cos(theta_2 + theta_3) - L_4*cos(theta_2 + theta_3 + theta_4))*sin(theta_2 + theta_3 + theta_4)*cos(theta_1)^2 - 1.0*L_4*m_3*(-L_3*cos(theta_2 + theta_3) - L_4*cos(theta_2 + theta_3 + theta_4))*sin(theta_1)^2*sin(theta_2 + theta_3 + theta_4) + 1.0*L_4*m_4*(-L_3*sin(theta_2 + theta_3) - L_4*sin(theta_2 + theta_3 + theta_4))*cos(theta_2 + theta_3 + theta_4)) + thetad_4*(1.0*L_4^2*m_2*sin(theta_2 + theta_3 + theta_4)*cos(theta_1)^2*cos(theta_2 + theta_3 + theta_4) + 1.0*L_4^2*m_3*sin(theta_1)^2*sin(theta_2 + theta_3 + theta_4)*cos(theta_2 + theta_3 + theta_4) - 1.0*L_4^2*m_4*sin(theta_2 + theta_3 + theta_4)*cos(theta_2 + theta_3 + theta_4));
C44 = thetad_1*(-1.0*L_4^2*m_2*sin(theta_1)*sin(theta_2 + theta_3 + theta_4)^2*cos(theta_1) + 1.0*L_4^2*m_3*sin(theta_1)*sin(theta_2 + theta_3 + theta_4)^2*cos(theta_1)) + thetad_2*(1.0*L_4^2*m_2*sin(theta_2 + theta_3 + theta_4)*cos(theta_1)^2*cos(theta_2 + theta_3 + theta_4) + 1.0*L_4^2*m_3*sin(theta_1)^2*sin(theta_2 + theta_3 + theta_4)*cos(theta_2 + theta_3 + theta_4) - 1.0*L_4^2*m_4*sin(theta_2 + theta_3 + theta_4)*cos(theta_2 + theta_3 + theta_4)) + thetad_3*(1.0*L_4^2*m_2*sin(theta_2 + theta_3 + theta_4)*cos(theta_1)^2*cos(theta_2 + theta_3 + theta_4) + 1.0*L_4^2*m_3*sin(theta_1)^2*sin(theta_2 + theta_3 + theta_4)*cos(theta_2 + theta_3 + theta_4) - 1.0*L_4^2*m_4*sin(theta_2 + theta_3 + theta_4)*cos(theta_2 + theta_3 + theta_4)) + thetad_4*(1.0*L_4^2*m_2*sin(theta_2 + theta_3 + theta_4)*cos(theta_1)^2*cos(theta_2 + theta_3 + theta_4) + 1.0*L_4^2*m_3*sin(theta_1)^2*sin(theta_2 + theta_3 + theta_4)*cos(theta_2 + theta_3 + theta_4) - 1.0*L_4^2*m_4*sin(theta_2 + theta_3 + theta_4)*cos(theta_2 + theta_3 + theta_4));


C = [C11 C12 C13 C14;...
    C21 C22 C23 C24; ...
    C31 C32 C33 C34; ...
    C41 C42 C43 C44];
% %%%%%%%%%%%%%%%%%%%%%%%%%%%%%%%%%%%%%%%%%%%%%%%%%%%%%%%%%%%%%%%%%%%%%%%%%%%%%%%%%%%%%%%%%%%%%%%%%%%%%%%%%%5defining the gravitational torque vector taug

taug1 = 4.905*a_1*m_1*cos(theta_1) + 9.81*m_2*(L_2*cos(theta_1 + theta_2)/2 + a_1*cos(theta_1)) + 9.81*m_3*(L_2*cos(theta_1 + theta_2) + L_3*cos(theta_1 + theta_2 + theta_3)/2 + a_1*cos(theta_1)) + 9.81*m_4*(L_2*cos(theta_1 + theta_2) + L_3*cos(theta_1 + theta_2 + theta_3) + L_4*cos(theta_1 + theta_2 + theta_3 + theta_4)/2 + a_1*cos(theta_1));
taug2 = 4.905*L_2*m_2*cos(theta_1 + theta_2) + 9.81*m_3*(L_2*cos(theta_1 + theta_2) + L_3*cos(theta_1 + theta_2 + theta_3)/2) + 9.81*m_4*(L_2*cos(theta_1 + theta_2) + L_3*cos(theta_1 + theta_2 + theta_3) + L_4*cos(theta_1 + theta_2 + theta_3 + theta_4)/2);
taug3 = 4.905*L_3*m_3*cos(theta_1 + theta_2 + theta_3) + 9.81*m_4*(L_3*cos(theta_1 + theta_2 + theta_3) + L_4*cos(theta_1 + theta_2 + theta_3 + theta_4)/2);
taug4 = 4.905*L_4*m_4*cos(theta_1 + theta_2 + theta_3 + theta_4);

taug = [taug1; ...
        taug2; ...
        taug3; ...
        taug4];


tau = Kp*thetaE + Kd*thetaEd+ M*thetarefdd +C*thetarefd + taug;

%

== matlab function hand_assembly_3test/MATLAB Function ==
  data: theta input; EE output
function EE = endEffector(theta)
theta_1 = theta(1);
theta_2 = theta(2);
theta_3 = theta(3);
theta_4 = theta(4);
d_1 = 0.04288;
L_2 = 0.057755;
L_3 = 0.057755;
L_4 =0.055798;
a_1 = 0.053311;


EE_x = cos(theta_1)*(L_4*cos(theta_2+theta_3+theta_4)+L_3*cos(theta_2+theta_3) + a_1);
EE_y = sin(L_4*cos(theta_2+theta_3+theta_4)+L_3*cos(theta_2+theta_3) + a_1);
EE_z = L_4*sin(theta_2+theta_3+theta_4)+L_3*sin(theta_2+theta_3) + d_1;
EE_phi = theta_1+theta_2+theta_3+theta_4;
EE = [EE_x; EE_y; EE_z; EE_phi];

== matlab function hand_assembly_3test/finger 3 ==
  data: detectedDebris input; waypoints output; timepoints output
function [waypoints, timepoints] = selectTrajectory(detectedDebris)


switch detectedDebris   %time points vv
    case 1 %bolt      1   2   3   4   5   6   7   8   9    10
        waypoints =[  0   0   0   0   0   0   0   0   0    0; ... %thetafref sidejoint 1
                      0  pi/2   pi/2   pi/2 pi/2  pi/2  pi/2  pi/2  pi/2  pi/2; ... %thetaref joint 2
                      0  pi/4   pi/4   pi/4 pi/4  pi/4  pi/4  pi/4  pi/4  pi/4; ... %thetaref joint 3
                      0  pi/4   pi/4   pi/4 pi/4  pi/4  pi/4  pi/4  pi/4  pi/4];    %thetaref joint 4
        timepoints = [0, 1, 2, 3, 4, 5, 6, 7, 8, 9]; 
    case 2 %flat     1    2    3    4    5    6    7    8    9    10
        waypoints = [0    0    0    0    0    0    0    0    0    0; ... %thetafref sidejoint 1
                     0    0    0    0    0    0    0    0    0    0; ... %thetaref joint 2
                     0    0    0    0    0    0    0    0    0    0; ... %thetaref joint 3
                     0    0    0    0    0    0    0    0    0    0];    %thetaref joint 4
        timepoints = [0, 1, 2, 3, 4, 5, 6, 7, 8, 9]; 
    
    case 3 %sphere 1    2    3    4    5    6    7    8    9    10
        waypoints = [0    0    0  0    0    0    0    0    0    0; ... %thetafref sidejoint 1
                     0    0    0    0   1.5 1.5 1.5 1.5 1.5 1.5; ... %thetaref joint 2
                     0    0    0    0   pi/5 pi/5 pi/5 pi/5 pi/5 pi/5; ... %thetaref joint 3
                     0    0    0    0   pi/5 pi/5 pi/5 pi/5 pi/5 pi/5];    %thetaref joint 4
        timepoints = [0, 1, 2, 3, 4, 5, 6, 7, 8, 9];

    case 4 %one at a time 1    2    3    4    5    6    7    8    9    10
        waypoints =      [0    0    0     0    0    0    0    0    0    0 ; ... %thetafref sidejoint 1
                          0    pi/3 pi/3    0    0    0    0    0    0    0 ; ... %thetaref joint 2
                          0    pi/3 pi/3    0    0    0    0    0    0    0 ; ... %thetaref joint 3
                          0    pi/3 pi/3    0    0    0    0    0    0    0 ];    %thetaref joint 4
        timepoints = [0, 1, 2, 3, 4, 5, 6, 7, 8, 9]; 
    otherwise 
        %unknown     1    2    3    4    5    6    7    8    9    10
        waypoints = [0    0    0    0    0    0    0    0    0    0; ... %thetafref sidejoint 1
                     0    0    0    0    0    0    0    0    0    0; ... %thetaref joint 2
                     0    0    0    0    0    0    0    0    0    0; ... %thetaref joint 3
                     0    0    0    0    0    0    0    0    0    0];    %thetaref joint 4
        timepoints = [0, 1, 2, 3, 4, 5, 6, 7, 8, 9];  
end
end
